simulink library "ManualMotor"  (R2018b)
settings: Solver=VariableStepAuto  StartTime=0.0  StopTime=10.0  RelTol=1e-3
undefined symbols (not defined in the file): Stateflow
libraries: DriveStraight x1
settings Model: Creator=Sjoerd  LastModifiedBy=nico

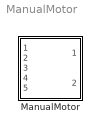
== system ManualMotor ==
  ManualMotor : Stateflow chart  TreatAsAtomicUnit=on

== stateflow chart ManualMotor/ManualMotor ==
  state StartStop
    (history)
    state Waiting
      entry:
      maxPower = 30
      rightMotor = 0
      leftMotor = 0
    state DriveStraight
    (default) -> Waiting
    Waiting -> DriveStraight : [SHORT_PRESS]
    DriveStraight -> Waiting : [after(500,msec) && SHORT_PRESS]
  state TurningRight
    entry:
    rightMotor = 0
    leftMotor = 30
  state TurningLEFT
    entry:
    rightMotor = 30
    leftMotor = 0
  (default) -> StartStop
  TurningRight -> StartStop : [RHOLD==false]
  TurningLEFT -> StartStop : [LHOLD==false]
  StartStop -> TurningRight [order 2] : [RHOLD]
  StartStop -> TurningLEFT [order 1] : [LHOLD]
  data: maxPower function_input; leftMotor output int32 size=1; rightMotor output int32 size=1; SHORT_PRESS input; RHOLD input; LHOLD input; leftEncoder input; rightEncoder input; maxPower local int32 size=1
